simulink model "SPGF_FSK_0000_R2019b"  (R2019b)
settings: Solver=ode3  SolverName=ode4  StartTime=0.0  StopTime=1.4  FixedStep=50e-6/50  RelTol=1e-3  EnableMultiTasking=on
undefined symbols (not defined in the file): D11, Delta
libraries: powerlib x2544, powerlib_meascontrol x204, simulink x24
(part 7 of 33)

== system SPGF_FSK_0000_R2019b/W60 ==
  DPL : Subsystem  Commented=on  mask{N=6, Frequency=[50], R_matrix=[0.347601410823579 0.0494303286168989 0.0494305228057156 0.0494305228057156 0.0494305228057156 0.0494305228057156;0.0494303286168989 0.63357380919679 0.0494305228057156 0.0494305228057156 0.0494305228057156 0.0494305228057156;0.0494305228057156 0.0494305228057156 0.347602052073771 0.0494309698670905 0.0494311641268522 0.0494311641268522;0.0494305228057156 0.0494305228057156 0.0494309698670905 0.633574450446981 0.0494311641268522 0.0494311641268522;0.0494305228057156 0.0494305228057156 0.0494311641268522 0.0494311641268522 0.347602052073771 0.0494309698670905;0.0494305228057156 0.0494305228057156 0.0494311641268522 0.0494311641268522 0.0494309698670905 0.633574450446981], L_matrix=[0.00260859879857304 0.00242332383525137 0.00221745883616686 0.00221745883616686 0.00221745883616686 0.00221745883616686;0.00242332383525137 0.00242198857850016 0.00221745883616686 0.00221745883616686 0.00221745883616686 0.00221745883616686;0.00221745883616686 0.00221745883616686 0.00253519514382882 0.00234992018050715 0.00223977112704788 0.00223977112704788;0.00221745883616686 0.00221745883616686 0.00234992018050715 0.00234858492375594 0.00223977112704788 0.00223977112704788;0.00221745883616686 0.00221745883616686 0.00223977112704788 0.00223977112704788 0.00253519514382882 0.00234992018050715;0.00221745883616686 0.00221745883616686 0.00223977112704788 0.00223977112704788 0.00234992018050715 0.00234858492375594], C_matrix=[1.90757475136094e-07 -1.90757475136094e-07 0 0 0 0;-1.90757475136094e-07 3.66052807704686e-07 0 0 0 0;0 0 1.90757475136094e-07 -1.90757475136094e-07 0 0;0 0 -1.90757475136094e-07 3.66052807704686e-07 0 0;0 0 0 0 1.90757475136094e-07 -1.90757475136094e-07;0 0 0 0 -1.90757475136094e-07 3.66052807704686e-07], Rg_matrix=[834331.357019417 -834331.357019417 Inf Inf Inf -Inf;-834331.357019417 434786.838789375 Inf Inf Inf -Inf;Inf Inf 834331.357019417 -834331.357019417 Inf -Inf;Inf Inf -834331.357019417 434786.838789375 Inf -Inf;Inf Inf Inf Inf 834331.357019417 -834331.357019417;Inf Inf Inf Inf -834331.357019417 434786.838789375], LineLength=[0.8]}
      mask prompts: N "Number of phases [N]"; Frequency "Frequency used for rlc specification [Hz]:"; R_matrix "Resistance per unit length [Ohms/km] NxN matrix"; L_matrix "Inductance per unit length [H/km] NxN matrix"; C_matrix "Capacitance per unit length [F/km] NxN matrix"; Rg_matrix "Resistance shunt matrix 6*6 [Ohm*km]"; LineLength "Line Length(km)"
      mask init:
      | % Rloss=1/(2*pi*Frequency*C_matrix(1,1)*TangLoss);
      | Rg_matrix=Rg_matrix./LineLength;
      mask Display:
      | port_label('lconn',1,'A');
      | port_label('lconn',2,'B');
      | port_label('lconn',3,'C');
      | 
      | port_label('rconn',1,'a');
      | port_label('rconn',2,'b');
      | port_label('rconn',3,'c');
      | 
      | disp('1x95');
  Pi : Subsystem  mask{R0=0.31, X0=0.083, Cp0=0.35, tg=2, Frequency=[50], LineLength=[0.8]}
      mask prompts: R0 "Удельное активное сопротивление, Ом/км"; X0 "Удельное индуктивное сопротивление, Ом/км"; Cp0 "Удельная рабочая емкость, мкФ/км"; tg "Тангенс диэлектрических потерь, %"; Frequency "Частота сети, Гц"; LineLength "Длина линии, км"
      mask init:
      | R=R0*LineLength;
      | L=X0*LineLength/(2*pi*Frequency);
      | Cp=Cp0*LineLength*1e-6;
      | Cmf=0.1525*Cp;
      | Cfg=0.56*Cp;
      | tg_pu=tg/100;
      | 
      | Rmf=1/(Cmf*2*pi*Frequency*tg_pu);
      | Rfg=1/(Cfg*2*pi*Frequency*tg_pu);
      mask Display:
      | port_label('lconn',1,'A');
      | port_label('lconn',2,'B');
      | port_label('lconn',3,'C');
      | 
      | port_label('rconn',1,'a');
      | port_label('rconn',2,'b');
      | port_label('rconn',3,'c');
      | 
      | disp('1x95');
  Q : Subsystem
  concentrated : Subsystem  Commented=on  mask{N=6, Frequency=[50], R_matrix=[0.347601410823579 0.0494303286168989 0.0494305228057156 0.0494305228057156 0.0494305228057156 0.0494305228057156;0.0494303286168989 0.63357380919679 0.0494305228057156 0.0494305228057156 0.0494305228057156 0.0494305228057156;0.0494305228057156 0.0494305228057156 0.347602052073771 0.0494309698670905 0.0494311641268522 0.0494311641268522;0.0494305228057156 0.0494305228057156 0.0494309698670905 0.633574450446981 0.0494311641268522 0.0494311641268522;0.0494305228057156 0.0494305228057156 0.0494311641268522 0.0494311641268522 0.347602052073771 0.0494309698670905;0.0494305228057156 0.0494305228057156 0.0494311641268522 0.0494311641268522 0.0494309698670905 0.633574450446981], L_matrix=[0.00260859879857304 0.00242332383525137 0.00221745883616686 0.00221745883616686 0.00221745883616686 0.00221745883616686;0.00242332383525137 0.00242198857850016 0.00221745883616686 0.00221745883616686 0.00221745883616686 0.00221745883616686;0.00221745883616686 0.00221745883616686 0.00253519514382882 0.00234992018050715 0.00223977112704788 0.00223977112704788;0.00221745883616686 0.00221745883616686 0.00234992018050715 0.00234858492375594 0.00223977112704788 0.00223977112704788;0.00221745883616686 0.00221745883616686 0.00223977112704788 0.00223977112704788 0.00253519514382882 0.00234992018050715;0.00221745883616686 0.00221745883616686 0.00223977112704788 0.00223977112704788 0.00234992018050715 0.00234858492375594], C_matrix=[1.90757475136094e-07 -1.90757475136094e-07 0 0 0 0;-1.90757475136094e-07 3.66052807704686e-07 0 0 0 0;0 0 1.90757475136094e-07 -1.90757475136094e-07 0 0;0 0 -1.90757475136094e-07 3.66052807704686e-07 0 0;0 0 0 0 1.90757475136094e-07 -1.90757475136094e-07;0 0 0 0 -1.90757475136094e-07 3.66052807704686e-07], Rg_matrix=[834331.357019417 -834331.357019417 Inf Inf Inf -Inf;-834331.357019417 434786.838789375 Inf Inf Inf -Inf;Inf Inf 834331.357019417 -834331.357019417 Inf -Inf;Inf Inf -834331.357019417 434786.838789375 Inf -Inf;Inf Inf Inf Inf 834331.357019417 -834331.357019417;Inf Inf Inf Inf -834331.357019417 434786.838789375], LineLength=[0.8]}
      mask prompts: N "Number of phases [N]"; Frequency "Frequency [Hz]:"; R_matrix "Resistance matrix 6*6 [Ohm/km]"; L_matrix "Inductance matrix 6*6 [H/km]"; C_matrix "Capacitance matrix 6*6 [F/km]"; Rg_matrix "Resistance shunt matrix 6*6 [Ohm*km]"; LineLength "Line Length(km)"
      mask init: same as SPGF_FSK_0000_R2019b/W11/concentrated
      mask Display:
      | port_label('lconn',1,'A');
      | port_label('lconn',2,'B');
      | port_label('lconn',3,'C');
      | 
      | port_label('rconn',1,'a');
      | port_label('rconn',2,'b');
      | port_label('rconn',3,'c');
      | 
      | disp('1x95');
  a : PMIOPort  Side=Right
  b : PMIOPort  Port=2  Side=Right
  c : PMIOPort  Port=3  Side=Right
  A : PMIOPort  Port=4  Side=Left
  B : PMIOPort  Port=5  Side=Left
  C : PMIOPort  Port=6  Side=Left
  connections:
  Pi/RConn2 -- Q/LConn2 -- concentrated/RConn2 -- DPL/RConn2
  Pi/RConn1 -- Q/LConn1 -- concentrated/RConn1 -- DPL/RConn1
  Pi/RConn3 -- Q/LConn3 -- concentrated/RConn3 -- DPL/RConn3
  Q/RConn2 -- b/RConn1
  Q/RConn1 -- a/RConn1
  Q/RConn3 -- c/RConn1
  DPL/LConn3 -- C/RConn1 -- Pi/LConn3 -- concentrated/LConn3
  concentrated/LConn2 -- B/RConn1 -- Pi/LConn2 -- DPL/LConn2
  concentrated/LConn1 -- A/RConn1 -- Pi/LConn1 -- DPL/LConn1

== system SPGF_FSK_0000_R2019b/W61 ==
  Q : Subsystem
  a : PMIOPort  Side=Right
  b : PMIOPort  Port=2  Side=Right
  c : PMIOPort  Port=3  Side=Right
  A : PMIOPort  Port=4  Side=Left
  B : PMIOPort  Port=5  Side=Left
  C : PMIOPort  Port=6  Side=Left
  connections:
  Q/RConn3 -- c/RConn1
  Q/RConn1 -- a/RConn1
  Q/RConn2 -- b/RConn1
  Q/LConn3 -- C/RConn1
  Q/LConn1 -- A/RConn1
  Q/LConn2 -- B/RConn1

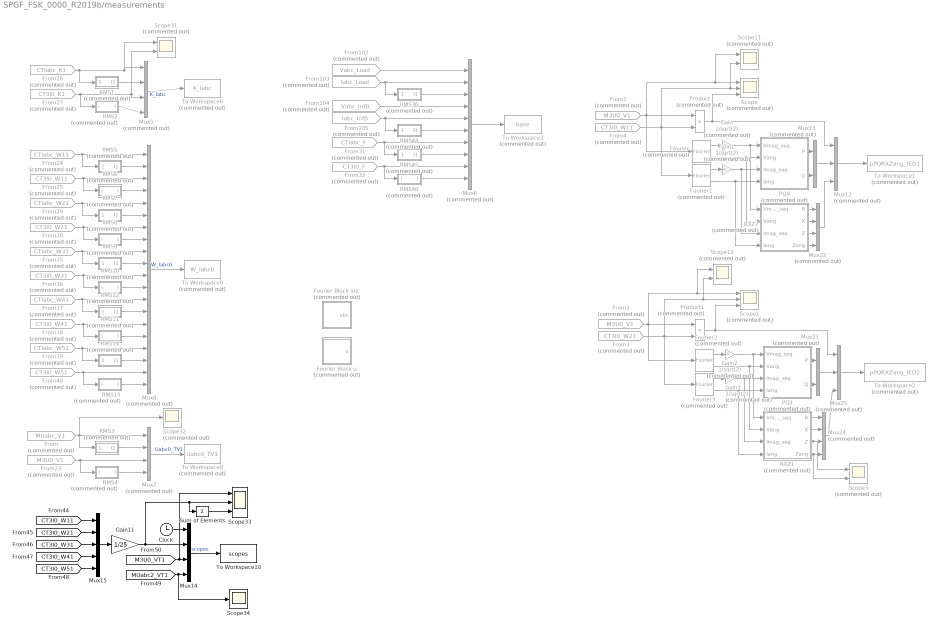
== system SPGF_FSK_0000_R2019b/measurements ==
  Clock : Clock
  Fourier{,1..3} (4 alike) : powerlib_meascontrol/Measurements/Fourier  Commented=on  Freq=50  n=1  InInit=[0, 0]  Ts=FTime
  Fourier Block abc : Subsystem  Commented=on
  Fourier Block u : Subsystem  Commented=on
  From : From  Commented=on  GotoTag=MUabc_V1  TagVisibility=global
  From1 : From  Commented=on  GotoTag=M3U0_V1  TagVisibility=global
  From102 : From  Commented=on  GotoTag=Vabc_Load  TagVisibility=global
  From103 : From  Commented=on  GotoTag=Iabc_Load  TagVisibility=global
  From104 : From  Commented=on  GotoTag=Vabc_InfB  TagVisibility=global
  From105 : From  Commented=on  GotoTag=Iabc_InfB  TagVisibility=global
  From2 : From  Commented=on  GotoTag=M3U0_V1  TagVisibility=global
  From23 : From  Commented=on  GotoTag=M3U0_V1  TagVisibility=global
  From24 : From  Commented=on  GotoTag=CTIabc_W11  TagVisibility=global
  From25 : From  Commented=on  GotoTag=CT3I0_W11  TagVisibility=global
  From26 : From  Commented=on  GotoTag=CTIabc_K1  TagVisibility=global
  From27 : From  Commented=on  GotoTag=CT3I0_K1  TagVisibility=global
  From29 : From  Commented=on  GotoTag=CTIabc_W21  TagVisibility=global
  From3 : From  Commented=on  GotoTag=CT3I0_W21  TagVisibility=global
  From30 : From  Commented=on  GotoTag=CT3I0_W21  TagVisibility=global
  From31 : From  Commented=on  GotoTag=CTIabc_F  TagVisibility=global
  From32 : From  Commented=on  GotoTag=CT3I0_F  TagVisibility=global
  From35 : From  Commented=on  GotoTag=CTIabc_W31  TagVisibility=global
  From36 : From  Commented=on  GotoTag=CT3I0_W31  TagVisibility=global
  From37 : From  Commented=on  GotoTag=CTIabc_W41  TagVisibility=global
  From38 : From  Commented=on  GotoTag=CT3I0_W41  TagVisibility=global
  From39 : From  Commented=on  GotoTag=CTIabc_W51  TagVisibility=global
  From4 : From  Commented=on  GotoTag=CT3I0_W11  TagVisibility=global
  From40 : From  Commented=on  GotoTag=CT3I0_W51  TagVisibility=global
  Gain{,1..3} (4 alike) : Gain  Commented=on  Gain=1/sqrt(2)
  Gain11 : Gain  Gain=1/25
  Mux12 : Mux  Commented=on  Inputs=3
  Mux13 : Mux  Commented=on  Inputs=2
  Mux14 : Mux
  Mux15 : Mux  Inputs=5
  Mux{5,7,22,24} (4 alike) : Mux  Commented=on
  Mux23 : Mux  Commented=on  Inputs=2
  Mux25 : Mux  Commented=on  Inputs=3
  Mux6 : Mux  Commented=on  Inputs=10
  Mux8 : Mux  Commented=on  Inputs=20
  PQ1 : Subsystem  Commented=on
  PQ8 : Subsystem  Commented=on
  Product : Product  Commented=on
  Product1 : Product  Commented=on
  RMS1 : Subsystem  Commented=on
  RMS10 : Subsystem  Commented=on
  RMS11 : Subsystem  Commented=on
  RMS12 : Subsystem  Commented=on
  RMS13 : Subsystem  Commented=on
  RMS14 : Subsystem  Commented=on
  RMS2 : Subsystem  Commented=on
  RMS3 : Subsystem  Commented=on
  RMS36 : Subsystem  Commented=on
  RMS4 : Subsystem  Commented=on
  RMS44 : Subsystem  Commented=on
  RMS45 : Subsystem  Commented=on
  RMS46 : Subsystem  Commented=on
  RMS5 : Subsystem  Commented=on
  RMS6 : Subsystem  Commented=on
  RMS7 : Subsystem  Commented=on
  RMS8 : Subsystem  Commented=on
  RMS9 : Subsystem  Commented=on
  RXZ1 : Subsystem  Commented=on
  RXZ7 : Subsystem  Commented=on
  Scope : Scope  Commented=on  NumInputPorts=3
  Scope1 : Scope  Commented=on  NumInputPorts=3
  Scope{3,11..12,31} (4 alike) : Scope  Commented=on  NumInputPorts=2
  Scope32 : Scope  Commented=on
  Scope33 : Scope  NumInputPorts=3
  Scope34 : Scope
  Sum of Elements : Sum  Inputs=+
  To Workspace1 : ToWorkspace  Commented=on  VariableName=pPQRXZang_IED1  SampleTime=-1
      settings: Save2DSignal=2-D array (concatenate along first dimension)
  To Workspace10 : ToWorkspace  VariableName=scopes  SampleTime=-1
      settings: Save2DSignal=2-D array (concatenate along first dimension)
  To Workspace2 : ToWorkspace  Commented=on  VariableName=pPQRXZang_IED2  SampleTime=-1
      settings: Save2DSignal=2-D array (concatenate along first dimension)
  To Workspace3 : ToWorkspace  Commented=on  VariableName=base  SaveFormat=Structure With Time  SampleTime=-1
      settings: Save2DSignal=2-D array (concatenate along first dimension)
  To Workspace6 : ToWorkspace  Commented=on  VariableName=K_Iabc  SampleTime=-1
      settings: Save2DSignal=2-D array (concatenate along first dimension)
  To Workspace8 : ToWorkspace  Commented=on  VariableName=Uabc0_TV1  SampleTime=-1
      settings: Save2DSignal=2-D array (concatenate along first dimension)
  To Workspace9 : ToWorkspace  Commented=on  VariableName=W_Iabc0  SampleTime=-1
      settings: Save2DSignal=2-D array (concatenate along first dimension)
  wires:
  From103/1 -> Mux6/2, RMS36/1(abc)
  From102/1 -> Mux6/1
  From104/1 -> Mux6/4
  From105/1 -> Mux6/5, RMS44/1(abc)
  From31/1 -> Mux6/7, RMS45/1(abc)
  From32/1 -> Mux6/9, RMS46/1(i)
  RMS36/1(I1) -> Mux6/3
  Mux6/1 -> To Workspace3/1
  RMS44/1(I1) -> Mux6/6
  RMS45/1(I1) -> Mux6/8
  RMS46/1(I) -> Mux6/10
  From4/1 -> Scope11/2, Scope/2, Fourier1/1, Product/2
  Product/1 -> Scope/3, Mux12/1
  Product1/1 -> Scope1/3, Mux25/1
  RXZ7/1(R) -> Mux22/1
  PQ8/2(Q) -> Mux13/2
  PQ8/1(P) -> Mux13/1
  RXZ7/2(X) -> Mux22/2
  RXZ7/4(Zang) -> Mux22/4
  Fourier/1 -> Gain/1
  Fourier1/2 -> RXZ7/4(Iang), PQ8/4(Iang)
  RXZ7/3(Z) -> Mux22/3
  Fourier1/1 -> Gain1/1
  Fourier/2 -> PQ8/2(Vang), RXZ7/2(Vang)
  Mux12/1 -> To Workspace1/1
  Gain/1 -> PQ8/1(Vmag_seq), RXZ7/1(Vmag_seq)
  Gain1/1 -> RXZ7/3(Imag_seq), PQ8/3(Imag_seq)
  Mux13/1 -> Mux12/2
  Mux22/1 -> Mux12/3
  From3/1 -> Scope1/2, Scope12/2, Fourier3/1, Product1/2
  From2/1 -> Scope12/1, Scope1/1, Fourier2/1, Product1/1
  RXZ1/1(R) -> Mux24/1
  PQ1/2(Q) -> Mux23/2
  PQ1/1(P) -> Mux23/1
  RXZ1/2(X) -> Mux24/2
  RXZ1/4(Zang) -> Scope3/2, Mux24/4
  Fourier2/1 -> Gain2/1
  Fourier3/2 -> PQ1/4(Iang), RXZ1/4(Iang)
  RXZ1/3(Z) -> Scope3/1, Mux24/3
  Fourier3/1 -> Gain3/1
  Fourier2/2 -> RXZ1/2(Vang), PQ1/2(Vang)
  Gain2/1 -> RXZ1/1(Vmag_seq), PQ1/1(Vmag_seq)
  Gain3/1 -> PQ1/3(Imag_seq), RXZ1/3(Imag_seq)
  Mux23/1 -> Mux25/2
  Mux24/1 -> Mux25/3
  Mux25/1 -> To Workspace2/1
  From1/1 -> Scope11/1, Scope/1, Fourier/1, Product/1
  From27/1 -> Scope31/2, Mux5/3, RMS2/1(i)
  From26/1 -> Scope31/1, Mux5/1, RMS1/1(abc)
  RMS1/1(I1) -> Mux5/2
  RMS2/1(I) -> Mux5/4
  Mux5/1 -> To Workspace6/1  "K_Iabc"
  Mux7/1 -> To Workspace8/1  "Uabc0_TV1"
  RMS4/1(I) -> Mux7/4
  RMS3/1(I1) -> Mux7/2
  From/1 -> Mux7/1, Scope32/1, RMS3/1(abc)
  From23/1 -> Mux7/3, RMS4/1(i)
  Mux8/1 -> To Workspace9/1  "W_Iabc0"
  RMS6/1(I) -> Mux8/4
  RMS5/1(I1) -> Mux8/2
  From24/1 -> RMS5/1(abc), Mux8/1
  From25/1 -> RMS6/1(i), Mux8/3
  From30/1 -> Mux8/7, RMS8/1(i)
  From29/1 -> Mux8/5, RMS7/1(abc)
  RMS7/1(I1) -> Mux8/6
  RMS8/1(I) -> Mux8/8
  RMS10/1(I) -> Mux8/12
  RMS9/1(I1) -> Mux8/10
  From35/1 -> Mux8/9, RMS9/1(abc)
  From36/1 -> Mux8/11, RMS10/1(i)
  From38/1 -> Mux8/15, RMS11/1(i)
  From37/1 -> Mux8/13, RMS12/1(abc)
  RMS12/1(I1) -> Mux8/14
  RMS11/1(I) -> Mux8/16
  RMS13/1(I) -> Mux8/20
  RMS14/1(I1) -> Mux8/18
  From39/1 -> Mux8/17, RMS14/1(abc)
  From40/1 -> Mux8/19, RMS13/1(i)
  Mux14/1 -> To Workspace10/1  "scopes"
  [CT3I0_W11] -> Mux15/1
  [CT3I0_W21] -> Mux15/2
  [CT3I0_W31] -> Mux15/3
  [CT3I0_W41] -> Mux15/4
  [CT3I0_W51] -> Mux15/5
  Mux15/1 -> Gain11/1
  Gain11/1 -> Mux14/2, Sum of Elements/1, Scope33/2
  [M3U0_VT1] -> Mux14/3, Scope33/1
  [MUabc2_VT1] -> Scope34/1, Mux14/4
  Clock/1 -> Mux14/1
  Sum of Elements/1 -> Scope33/3

== system SPGF_FSK_0000_R2019b/Feed/Q ==
  breaker : Subsystem  Commented=on  mask{SwitchA=off, SwitchB=off, SwitchC=off, InitialStatus=[1 1 1], BreakerResistance=0.0001, SnubberResistance=1e6, SnubberCapacitance=inf, TransitionTimes=[0.5 0.7], ShiftTimes=[0 0 0]}
      mask prompts: SwitchA "Switching of phase A"; SwitchB "Switching of phase B"; SwitchC "Switching of phase C"; InitialStatus "Initial status of phase breaker [A, B, C]"; BreakerResistance "Breaker resistance Ron (ohms) :"; SnubberResistance "Snubbers resistance Rp (ohms) :"; SnubberCapacitance "Snubbers capacitance Cp (F) :"; TransitionTimes "Transition times (s) :"; ShiftTimes "Time differences for switch [tA, tB, tC] (s) :"
      mask init:
      | SwitchA = double(SwitchA);
      | SwitchB = double(SwitchB);
      | SwitchC = double(SwitchC);
      | SwitchStatusA(1) = double((logical(InitialStatus(1))));
      | SwitchStatusB(1) = double((logical(InitialStatus(2))));
      | SwitchStatusC(1) = double((logical(InitialStatus(3))));
      | for i=1:length(TransitionTimes)
      |     SwitchStatusA(i+1) = double(~(logical(SwitchStatusA(i))));
      |     SwitchStatusB(i+1) = double(~(logical(SwitchStatusB(i))));
      |     SwitchStatusC(i+1) = double(~(logical(SwitchStatusC(i))));
      | end
      | SwitchTimesA = [0,TransitionTimes+ShiftTimes(1)];
      | SwitchTimesB = [0,TransitionTimes+ShiftTimes(2)];
      | SwitchTimesC = [0,TransitionTimes+ShiftTimes(3)];
      mask Display:
      | % port_label('input',1,'Iabc');
      | 
      | port_label('lconn',1,'A');
      | port_label('lconn',2,'B');
      | port_label('lconn',3,'C');
      | 
      | port_label('rconn',1,'a');
      | port_label('rconn',2,'b');
      | port_label('rconn',3,'c');
      | 
      | disp('   Q    ');
  meas : Subsystem
  shunt : Subsystem
  A : PMIOPort  Side=Right
  B : PMIOPort  Port=2  Side=Right
  C : PMIOPort  Port=3  Side=Right
  a : PMIOPort  Port=4  Side=Left
  b : PMIOPort  Port=5  Side=Left
  c : PMIOPort  Port=6  Side=Left
  connections:
  breaker/RConn1 -- meas/LConn1 -- shunt/RConn1
  breaker/RConn2 -- meas/LConn2 -- shunt/RConn2
  shunt/RConn3 -- breaker/RConn3 -- meas/LConn3
  shunt/LConn3 -- C/RConn1 -- breaker/LConn3
  shunt/LConn1 -- A/RConn1 -- breaker/LConn1
  shunt/LConn2 -- B/RConn1 -- breaker/LConn2
  meas/RConn1 -- a/RConn1
  meas/RConn2 -- b/RConn1
  meas/RConn3 -- c/RConn1

== system SPGF_FSK_0000_R2019b/Harmonic/Fourier Block1 ==
  in : Inport
  Display : Display
  Fourier : powerlib_meascontrol/Measurements/Fourier  Freq=50  n=1  InInit=[0, 0]  Ts=0
  Fourier1 : powerlib_meascontrol/Measurements/Fourier  Freq=50  n=2  InInit=[0, 0]  Ts=0
  Fourier2 : powerlib_meascontrol/Measurements/Fourier  Freq=50  n=3  InInit=[0, 0]  Ts=0
  Fourier3 : powerlib_meascontrol/Measurements/Fourier  Freq=50  n=5  InInit=[0, 0]  Ts=0
  Fourier4 : powerlib_meascontrol/Measurements/Fourier  Freq=50  n=7  InInit=[0, 0]  Ts=0
  Fourier5 : powerlib_meascontrol/Measurements/Fourier  Freq=50  n=9  InInit=[0, 0]  Ts=0
  Fourier6 : powerlib_meascontrol/Measurements/Fourier  Freq=50  n=11  InInit=[0, 0]  Ts=0
  Fourier7 : powerlib_meascontrol/Measurements/Fourier  Freq=50  n=13  InInit=[0, 0]  Ts=0
  Fourier8 : powerlib_meascontrol/Measurements/Fourier  Freq=50  n=15  InInit=[0, 0]  Ts=0
  Fourier9 : powerlib_meascontrol/Measurements/Fourier  Freq=50  n=17  InInit=[0, 0]  Ts=0
  Mux : Mux  Inputs=10
  Scope{2..11} (10 alike) : Scope
  Terminator{,1..9} (10 alike) : Terminator
  wires:
  Mux/1 -> Display/1
  Fourier5/1 -> Scope7/1, Mux/6
  Fourier4/1 -> Scope6/1, Mux/5
  Fourier3/1 -> Scope5/1, Mux/4
  in/1 -> Fourier/1, Fourier1/1, Fourier2/1, Fourier3/1, Fourier4/1, Fourier5/1, Fourier6/1, Fourier7/1, Fourier8/1, Fourier9/1
  Fourier1/1 -> Mux/2, Scope3/1
  Fourier9/2 -> Terminator9/1
  Fourier2/1 -> Scope4/1, Mux/3
  Fourier/1 -> Mux/1, Scope2/1
  Fourier3/2 -> Terminator5/1
  Fourier4/2 -> Terminator4/1
  Fourier5/2 -> Terminator3/1
  Fourier1/2 -> Terminator1/1
  Fourier/2 -> Terminator2/1
  Fourier8/2 -> Terminator6/1
  Fourier6/2 -> Terminator8/1
  Fourier7/2 -> Terminator7/1
  Fourier2/2 -> Terminator/1
  Fourier9/1 -> Scope11/1, Mux/10
  Fourier6/1 -> Scope8/1, Mux/7
  Fourier8/1 -> Scope10/1, Mux/9
  Fourier7/1 -> Scope9/1, Mux/8

== system SPGF_FSK_0000_R2019b/Harmonic/Fourier Block2 ==
  in : Inport
  Display : Display
  Fourier : powerlib_meascontrol/Measurements/Fourier  Freq=50  n=1  InInit=[0, 0]  Ts=0
  Fourier1 : powerlib_meascontrol/Measurements/Fourier  Freq=50  n=2  InInit=[0, 0]  Ts=0
  Fourier2 : powerlib_meascontrol/Measurements/Fourier  Freq=50  n=3  InInit=[0, 0]  Ts=0
  Fourier3 : powerlib_meascontrol/Measurements/Fourier  Freq=50  n=5  InInit=[0, 0]  Ts=0
  Fourier4 : powerlib_meascontrol/Measurements/Fourier  Freq=50  n=7  InInit=[0, 0]  Ts=0
  Fourier5 : powerlib_meascontrol/Measurements/Fourier  Freq=50  n=9  InInit=[0, 0]  Ts=0
  Fourier6 : powerlib_meascontrol/Measurements/Fourier  Freq=50  n=11  InInit=[0, 0]  Ts=0
  Fourier7 : powerlib_meascontrol/Measurements/Fourier  Freq=50  n=13  InInit=[0, 0]  Ts=0
  Fourier8 : powerlib_meascontrol/Measurements/Fourier  Freq=50  n=15  InInit=[0, 0]  Ts=0
  Fourier9 : powerlib_meascontrol/Measurements/Fourier  Freq=50  n=17  InInit=[0, 0]  Ts=0
  Mux : Mux  Inputs=10
  Scope{2..11} (10 alike) : Scope
  Terminator{,1..9} (10 alike) : Terminator
  wires:
  Fourier7/1 -> Mux/8, Scope9/1
  Fourier8/1 -> Mux/9, Scope10/1
  Fourier6/1 -> Mux/7, Scope8/1
  Fourier9/1 -> Mux/10, Scope11/1
  Fourier2/2 -> Terminator/1
  Fourier7/2 -> Terminator7/1
  Fourier6/2 -> Terminator8/1
  Fourier8/2 -> Terminator6/1
  Fourier/2 -> Terminator2/1
  Fourier1/2 -> Terminator1/1
  Fourier5/2 -> Terminator3/1
  Fourier4/2 -> Terminator4/1
  Fourier3/2 -> Terminator5/1
  Fourier/1 -> Scope2/1, Mux/1
  Fourier2/1 -> Mux/3, Scope4/1
  Fourier9/2 -> Terminator9/1
  Fourier1/1 -> Scope3/1, Mux/2
  in/1 -> Fourier9/1, Fourier8/1, Fourier7/1, Fourier6/1, Fourier5/1, Fourier4/1, Fourier3/1, Fourier2/1, Fourier1/1, Fourier/1
  Fourier3/1 -> Mux/4, Scope5/1
  Fourier4/1 -> Mux/5, Scope6/1
  Fourier5/1 -> Mux/6, Scope7/1
  Mux/1 -> Display/1

== system SPGF_FSK_0000_R2019b/Harmonic/Subsystem1 ==
  clock : Inport
  phase : Inport  Port=2
  Add : Sum
  Add1 : Sum
  Constant1 : Constant  Value=HN
  Constant2 : Constant  Value=Percent./100
  Constant3 : Constant  Value=PhaseH
  Dot Product : DotProduct  OutDataTypeStr=double  RndMeth=Nearest  InputSameDT=on
  Product15 : Product
  Trigonometric Function : Trigonometry  Operator=cos
  amp : Gain  Gain=Current*sqrt(2)
  deg2rad : Gain  Gain=pi/180
  omega1 : Gain  Gain=2*pi*Frequency
  o : Outport
  wires:
  Constant3/1 -> Add1/1
  Product15/1 -> Add/1
  deg2rad/1 -> Add/2
  phase/1 -> Add1/2
  Dot Product/1 -> o/1
  Add/1 -> Trigonometric Function/1
  Trigonometric Function/1 -> Dot Product/2
  clock/1 -> Product15/2
  Constant1/1 -> omega1/1
  Add1/1 -> deg2rad/1
  Constant2/1 -> amp/1
  amp/1 -> Dot Product/1
  omega1/1 -> Product15/1

== system SPGF_FSK_0000_R2019b/Harmonic/Subsystem2 ==
  clock : Inport
  phase : Inport  Port=2
  Add : Sum
  Add1 : Sum
  Constant1 : Constant  Value=HN
  Constant2 : Constant  Value=Percent./100
  Constant3 : Constant  Value=PhaseH
  Dot Product : DotProduct  OutDataTypeStr=double  RndMeth=Nearest  InputSameDT=on
  Product15 : Product
  Trigonometric Function : Trigonometry  Operator=cos
  amp : Gain  Gain=Current*sqrt(2)
  deg2rad : Gain  Gain=pi/180
  omega1 : Gain  Gain=2*pi*Frequency
  o : Outport
  wires:
  omega1/1 -> Product15/1
  amp/1 -> Dot Product/1
  Constant2/1 -> amp/1
  Add1/1 -> deg2rad/1
  Constant1/1 -> omega1/1
  clock/1 -> Product15/2
  Trigonometric Function/1 -> Dot Product/2
  Add/1 -> Trigonometric Function/1
  Dot Product/1 -> o/1
  phase/1 -> Add1/2
  deg2rad/1 -> Add/2
  Product15/1 -> Add/1
  Constant3/1 -> Add1/1

== system SPGF_FSK_0000_R2019b/Harmonic/Subsystem3 ==
  clock : Inport
  phase : Inport  Port=2
  Add : Sum
  Add1 : Sum
  Constant1 : Constant  Value=HN
  Constant2 : Constant  Value=Percent./100
  Constant3 : Constant  Value=PhaseH
  Dot Product : DotProduct  OutDataTypeStr=double  RndMeth=Nearest  InputSameDT=on
  Product15 : Product
  Trigonometric Function : Trigonometry  Operator=cos
  amp : Gain  Gain=Current*sqrt(2)
  deg2rad : Gain  Gain=pi/180
  omega1 : Gain  Gain=2*pi*Frequency
  o : Outport
  wires:
  omega1/1 -> Product15/1
  amp/1 -> Dot Product/1
  Constant2/1 -> amp/1
  Add1/1 -> deg2rad/1
  Constant1/1 -> omega1/1
  clock/1 -> Product15/2
  Trigonometric Function/1 -> Dot Product/2
  Add/1 -> Trigonometric Function/1
  Dot Product/1 -> o/1
  phase/1 -> Add1/2
  deg2rad/1 -> Add/2
  Product15/1 -> Add/1
  Constant3/1 -> Add1/1

== system SPGF_FSK_0000_R2019b/K1/fault ==
  Add : Sum  Inputs=+-
  Arcing : Subsystem  TreatAsAtomicUnit=on
  Constant2 : Constant  Value=FaultPhase
  Control : Product  Inputs=***
  Count Limiter : Subsystem
  Demux : Demux  Outputs=2
  Fault Interruption : Subsystem
  Fault A : Constant  Value=FaultA
  Fault A1 : Constant  Value=0
  Fault A2 : Constant  Value=LimitArcNum
  Fault A3 : Constant  Value=AddTimeDelay
  Fault B : Constant  Value=FaultB
  Fault C : Constant  Value=FaultC
  Ground1 : powerlib/Elements/Ground  LConnTagsString=a
  Ideal Switch A : powerlib/Power Electronics/Ideal Switch  Ron=FaultResistance  Lon=0  IC=0  Rs=SnubberResistance  Cs=SnubberCapacitance  Measurements=on
  Ideal Switch B : powerlib/Power Electronics/Ideal Switch  Ron=FaultResistance  Lon=0  IC=0  Rs=SnubberResistance  Cs=SnubberCapacitance  Measurements=on
  Ideal Switch C : powerlib/Power Electronics/Ideal Switch  Ron=FaultResistance  Lon=0  IC=0  Rs=SnubberResistance  Cs=SnubberCapacitance  Measurements=on
  Mux : Mux  Inputs=2
  Product : Product
  Product1 : Product
  Product2 : Product
  Rground : powerlib/Elements/Series RLC Branch  LConnTagsString=__new0  RConnTagsString=__new0  BranchType=R  Resistance=GroundResistance  Inductance=0  SetiL0=off  InitialCurrent=0  Capacitance=inf  Setx0=off  InitialVoltage=0  Measurements=None
  SW : MultiPortSwitch  DataPortForDefault=Additional data port
  SW_Limit : Switch  Criteria=u2 > Threshold  Threshold=0.5
  SW_TD : Switch  Criteria=u2 > Threshold  Threshold=0.5
  Step : Step  Time=EndFaultTime  SampleTime=0
  Step1 : Step  Time=BeginFaultTime  SampleTime=0
  Time Delay : Subsystem
  A : PMIOPort  Side=Left
  B : PMIOPort  Port=2  Side=Left
  C : PMIOPort  Port=3  Side=Left
  wires:
  Demux/2 -> [V]
  Time Delay/1(O) -> SW_TD/1
  Count Limiter/1(Count) -> Time Delay/1(Count)
  SW_TD/1 -> Count Limiter/1(I), SW_Limit/3
  Fault A3/1 -> SW_TD/2
  SW_Limit/1 -> Product2/1, Product1/1, Product/1
  Fault Interruption/1(O) -> Control/3
  Constant2/1 -> SW/1
  SW/1 -> Demux/1
  Fault A1/1 -> SW/5
  Ideal Switch A/1 -> SW/2
  Ideal Switch B/1 -> SW/3
  Ideal Switch C/1 -> SW/4
  Fault A/1 -> Product/2
  Product/1 -> Ideal Switch A/1
  Fault B/1 -> Product1/2
  Product1/1 -> Ideal Switch B/1
  Fault C/1 -> Product2/2
  Product2/1 -> Ideal Switch C/1
  Step1/1 -> Add/1
  Step/1 -> Add/2
  Add/1 -> Arcing/Enable, Control/1
  [I] -> Mux/1
  [V] -> Mux/2
  Mux/1 -> Arcing/1(I)
  Arcing/1(O) -> Control/2
  Fault A2/1 -> SW_Limit/2
  Count Limiter/2(O) -> SW_Limit/1
  Control/1 -> SW_TD/3, Time Delay/2(Control)
  Demux/1 -> [I]
  connections:
  Ideal Switch C/LConn1 -- C/RConn1
  Ideal Switch A/LConn1 -- A/RConn1
  Ideal Switch B/LConn1 -- B/RConn1
  Ideal Switch C/RConn1 -- Rground/LConn1 -- Ideal Switch A/RConn1 -- Ideal Switch B/RConn1
  Ground1/LConn1 -- Rground/RConn1

== system SPGF_FSK_0000_R2019b/K1/meas ==
  Add : Sum  Inputs=+++
  GainI : Gain
  GainI0 : Gain
  I A: : powerlib/Measurements/Current Measurement  PhasorSimulation=off  OutputType=Complex  PSBequivalent=0
  I B: : powerlib/Measurements/Current Measurement  PhasorSimulation=off  OutputType=Complex  PSBequivalent=0
  I C: : powerlib/Measurements/Current Measurement  PhasorSimulation=off  OutputType=Complex  PSBequivalent=0
  Mux : Mux  Inputs=3
  A : PMIOPort  Side=Left
  B : PMIOPort  Port=2  Side=Left
  C : PMIOPort  Port=3  Side=Left
  a : PMIOPort  Port=4  Side=Right
  b : PMIOPort  Port=5  Side=Right
  c : PMIOPort  Port=6  Side=Right
  tag scope: CT3I0_K1=global, CTIabc_K1=global
  wires:
  GainI/1 -> [CTIabc_K1]
  Mux/1 -> GainI/1
  GainI0/1 -> [CT3I0_K1]
  Add/1 -> GainI0/1
  I C:/1 -> Add/3, Mux/3
  I B:/1 -> Add/2, Mux/2
  I A:/1 -> Add/1, Mux/1
  connections:
  I B:/LConn1 -- B/RConn1
  I C:/LConn1 -- C/RConn1
  I A:/LConn1 -- A/RConn1
  a/RConn1 -- I A:/RConn1
  I B:/RConn1 -- b/RConn1
  I C:/RConn1 -- c/RConn1

== system SPGF_FSK_0000_R2019b/K2/fault ==
  Add : Sum  Inputs=+-
  Arcing : Subsystem  TreatAsAtomicUnit=on
  Constant2 : Constant  Value=FaultPhase
  Control : Product  Inputs=***
  Count Limiter : Subsystem
  Demux : Demux  Outputs=2
  Fault Interruption : Subsystem
  Fault A : Constant  Value=FaultA
  Fault A1 : Constant  Value=0
  Fault A2 : Constant  Value=LimitArcNum
  Fault A3 : Constant  Value=AddTimeDelay
  Fault B : Constant  Value=FaultB
  Fault C : Constant  Value=FaultC
  Ground1 : powerlib/Elements/Ground  LConnTagsString=a
  Ideal Switch A : powerlib/Power Electronics/Ideal Switch  Ron=FaultResistance  Lon=0  IC=0  Rs=SnubberResistance  Cs=SnubberCapacitance  Measurements=on
  Ideal Switch B : powerlib/Power Electronics/Ideal Switch  Ron=FaultResistance  Lon=0  IC=0  Rs=SnubberResistance  Cs=SnubberCapacitance  Measurements=on
  Ideal Switch C : powerlib/Power Electronics/Ideal Switch  Ron=FaultResistance  Lon=0  IC=0  Rs=SnubberResistance  Cs=SnubberCapacitance  Measurements=on
  Mux : Mux  Inputs=2
  Product : Product
  Product1 : Product
  Product2 : Product
  Rground : powerlib/Elements/Series RLC Branch  LConnTagsString=__new0  RConnTagsString=__new0  BranchType=R  Resistance=GroundResistance  Inductance=0  SetiL0=off  InitialCurrent=0  Capacitance=inf  Setx0=off  InitialVoltage=0  Measurements=None
  SW : MultiPortSwitch  DataPortForDefault=Additional data port
  SW_Limit : Switch  Criteria=u2 > Threshold  Threshold=0.5
  SW_TD : Switch  Criteria=u2 > Threshold  Threshold=0.5
  Scope : Scope
  Step : Step  Time=EndFaultTime  SampleTime=0
  Step1 : Step  Time=BeginFaultTime  SampleTime=0
  Time Delay : Subsystem
  A : PMIOPort  Side=Left
  B : PMIOPort  Port=2  Side=Left
  C : PMIOPort  Port=3  Side=Left
  wires:
  Demux/2 -> [V]
  Time Delay/1(O) -> SW_TD/1
  Count Limiter/1(Count) -> Time Delay/1(Count)
  SW_TD/1 -> Count Limiter/1(I), SW_Limit/3
  Fault A3/1 -> SW_TD/2
  SW_Limit/1 -> Product2/1, Product1/1, Product/1
  Fault Interruption/1(O) -> Control/3
  Constant2/1 -> SW/1
  SW/1 -> Demux/1
  Fault A1/1 -> SW/5
  Ideal Switch A/1 -> SW/2
  Ideal Switch B/1 -> SW/3
  Ideal Switch C/1 -> SW/4
  Fault A/1 -> Product/2
  Product/1 -> Ideal Switch A/1
  Fault B/1 -> Product1/2
  Product1/1 -> Ideal Switch B/1
  Fault C/1 -> Product2/2
  Product2/1 -> Ideal Switch C/1
  Step1/1 -> Add/1
  Step/1 -> Add/2
  Add/1 -> Arcing/Enable, Control/1
  [I] -> Mux/1
  [V] -> Mux/2
  Mux/1 -> Arcing/1(I)
  Arcing/1(O) -> Control/2
  Fault A2/1 -> SW_Limit/2
  Count Limiter/2(O) -> SW_Limit/1
  Control/1 -> SW_TD/3, Time Delay/2(Control)
  Demux/1 -> Scope/1, [I]
  connections:
  Ideal Switch C/LConn1 -- C/RConn1
  Ideal Switch A/LConn1 -- A/RConn1
  Ideal Switch B/LConn1 -- B/RConn1
  Ideal Switch C/RConn1 -- Rground/LConn1 -- Ideal Switch A/RConn1 -- Ideal Switch B/RConn1
  Ground1/LConn1 -- Rground/RConn1

== system SPGF_FSK_0000_R2019b/K2/meas ==
  Add : Sum  Inputs=+++
  GainI : Gain
  GainI0 : Gain
  I A: : powerlib/Measurements/Current Measurement  PhasorSimulation=off  OutputType=Complex  PSBequivalent=0
  I B: : powerlib/Measurements/Current Measurement  PhasorSimulation=off  OutputType=Complex  PSBequivalent=0
  I C: : powerlib/Measurements/Current Measurement  PhasorSimulation=off  OutputType=Complex  PSBequivalent=0
  Mux : Mux  Inputs=3
  A : PMIOPort  Side=Left
  B : PMIOPort  Port=2  Side=Left
  C : PMIOPort  Port=3  Side=Left
  a : PMIOPort  Port=4  Side=Right
  b : PMIOPort  Port=5  Side=Right
  c : PMIOPort  Port=6  Side=Right
  tag scope: CT3I0_K2=global, CTIabc_K2=global
  wires:
  I A:/1 -> Mux/1, Add/1
  I B:/1 -> Mux/2, Add/2
  I C:/1 -> Mux/3, Add/3
  Add/1 -> GainI0/1
  GainI0/1 -> [CT3I0_K2]
  Mux/1 -> GainI/1
  GainI/1 -> [CTIabc_K2]
  connections:
  I C:/RConn1 -- c/RConn1
  I B:/RConn1 -- b/RConn1
  a/RConn1 -- I A:/RConn1
  I A:/LConn1 -- A/RConn1
  I C:/LConn1 -- C/RConn1
  I B:/LConn1 -- B/RConn1

== system SPGF_FSK_0000_R2019b/K3/fault ==
  Add : Sum  Inputs=+-
  Arcing : Subsystem  TreatAsAtomicUnit=on
  Constant2 : Constant  Value=FaultPhase
  Control : Product  Inputs=***
  Count Limiter : Subsystem
  Demux : Demux  Outputs=2
  Fault Interruption : Subsystem
  Fault A : Constant  Value=FaultA
  Fault A1 : Constant  Value=0
  Fault A2 : Constant  Value=LimitArcNum
  Fault A3 : Constant  Value=AddTimeDelay
  Fault B : Constant  Value=FaultB
  Fault C : Constant  Value=FaultC
  Ground1 : powerlib/Elements/Ground  LConnTagsString=a
  Ideal Switch A : powerlib/Power Electronics/Ideal Switch  Ron=FaultResistance  Lon=0  IC=0  Rs=SnubberResistance  Cs=SnubberCapacitance  Measurements=on
  Ideal Switch B : powerlib/Power Electronics/Ideal Switch  Ron=FaultResistance  Lon=0  IC=0  Rs=SnubberResistance  Cs=SnubberCapacitance  Measurements=on
  Ideal Switch C : powerlib/Power Electronics/Ideal Switch  Ron=FaultResistance  Lon=0  IC=0  Rs=SnubberResistance  Cs=SnubberCapacitance  Measurements=on
  Mux : Mux  Inputs=2
  Product : Product
  Product1 : Product
  Product2 : Product
  Rground : powerlib/Elements/Series RLC Branch  LConnTagsString=__new0  RConnTagsString=__new0  BranchType=R  Resistance=GroundResistance  Inductance=0  SetiL0=off  InitialCurrent=0  Capacitance=inf  Setx0=off  InitialVoltage=0  Measurements=None
  SW : MultiPortSwitch  DataPortForDefault=Additional data port
  SW_Limit : Switch  Criteria=u2 > Threshold  Threshold=0.5
  SW_TD : Switch  Criteria=u2 > Threshold  Threshold=0.5
  Step : Step  Time=EndFaultTime  SampleTime=0
  Step1 : Step  Time=BeginFaultTime  SampleTime=0
  Time Delay : Subsystem
  A : PMIOPort  Side=Left
  B : PMIOPort  Port=2  Side=Left
  C : PMIOPort  Port=3  Side=Left
  wires:
  Demux/2 -> [V]
  Time Delay/1(O) -> SW_TD/1
  Count Limiter/1(Count) -> Time Delay/1(Count)
  SW_TD/1 -> Count Limiter/1(I), SW_Limit/3
  Fault A3/1 -> SW_TD/2
  SW_Limit/1 -> Product2/1, Product1/1, Product/1
  Fault Interruption/1(O) -> Control/3
  Constant2/1 -> SW/1
  SW/1 -> Demux/1
  Fault A1/1 -> SW/5
  Ideal Switch A/1 -> SW/2
  Ideal Switch B/1 -> SW/3
  Ideal Switch C/1 -> SW/4
  Fault A/1 -> Product/2
  Product/1 -> Ideal Switch A/1
  Fault B/1 -> Product1/2
  Product1/1 -> Ideal Switch B/1
  Fault C/1 -> Product2/2
  Product2/1 -> Ideal Switch C/1
  Step1/1 -> Add/1
  Step/1 -> Add/2
  Add/1 -> Arcing/Enable, Control/1
  [I] -> Mux/1
  [V] -> Mux/2
  Mux/1 -> Arcing/1(I)
  Arcing/1(O) -> Control/2
  Fault A2/1 -> SW_Limit/2
  Count Limiter/2(O) -> SW_Limit/1
  Control/1 -> SW_TD/3, Time Delay/2(Control)
  Demux/1 -> [I]
  connections:
  Ideal Switch C/LConn1 -- C/RConn1
  Ideal Switch A/LConn1 -- A/RConn1
  Ideal Switch B/LConn1 -- B/RConn1
  Ideal Switch C/RConn1 -- Rground/LConn1 -- Ideal Switch A/RConn1 -- Ideal Switch B/RConn1
  Ground1/LConn1 -- Rground/RConn1

== system SPGF_FSK_0000_R2019b/K3/meas ==
  Add : Sum  Inputs=+++
  GainI : Gain
  GainI0 : Gain
  I A: : powerlib/Measurements/Current Measurement  PhasorSimulation=off  OutputType=Complex  PSBequivalent=0
  I B: : powerlib/Measurements/Current Measurement  PhasorSimulation=off  OutputType=Complex  PSBequivalent=0
  I C: : powerlib/Measurements/Current Measurement  PhasorSimulation=off  OutputType=Complex  PSBequivalent=0
  Mux : Mux  Inputs=3
  A : PMIOPort  Side=Left
  B : PMIOPort  Port=2  Side=Left
  C : PMIOPort  Port=3  Side=Left
  a : PMIOPort  Port=4  Side=Right
  b : PMIOPort  Port=5  Side=Right
  c : PMIOPort  Port=6  Side=Right
  tag scope: CT3I0_K1=global, CTIabc_K1=global
  wires:
  I A:/1 -> Mux/1, Add/1
  I B:/1 -> Mux/2, Add/2
  I C:/1 -> Mux/3, Add/3
  Add/1 -> GainI0/1
  GainI0/1 -> [CT3I0_K1]
  Mux/1 -> GainI/1
  GainI/1 -> [CTIabc_K1]
  connections:
  I C:/RConn1 -- c/RConn1
  I B:/RConn1 -- b/RConn1
  a/RConn1 -- I A:/RConn1
  I A:/LConn1 -- A/RConn1
  I C:/LConn1 -- C/RConn1
  I B:/LConn1 -- B/RConn1

== system SPGF_FSK_0000_R2019b/K4/fault ==
  Add : Sum  Inputs=+-
  Arcing : Subsystem  TreatAsAtomicUnit=on
  Constant2 : Constant  Value=FaultPhase
  Control : Product  Inputs=***
  Count Limiter : Subsystem
  Demux : Demux  Outputs=2
  Fault Interruption : Subsystem
  Fault A : Constant  Value=FaultA
  Fault A1 : Constant  Value=0
  Fault A2 : Constant  Value=LimitArcNum
  Fault A3 : Constant  Value=AddTimeDelay
  Fault B : Constant  Value=FaultB
  Fault C : Constant  Value=FaultC
  Ground1 : powerlib/Elements/Ground  LConnTagsString=a
  Ideal Switch A : powerlib/Power Electronics/Ideal Switch  Ron=FaultResistance  Lon=0  IC=0  Rs=SnubberResistance  Cs=SnubberCapacitance  Measurements=on
  Ideal Switch B : powerlib/Power Electronics/Ideal Switch  Ron=FaultResistance  Lon=0  IC=0  Rs=SnubberResistance  Cs=SnubberCapacitance  Measurements=on
  Ideal Switch C : powerlib/Power Electronics/Ideal Switch  Ron=FaultResistance  Lon=0  IC=0  Rs=SnubberResistance  Cs=SnubberCapacitance  Measurements=on
  Mux : Mux  Inputs=2
  Product : Product
  Product1 : Product
  Product2 : Product
  Rground : powerlib/Elements/Series RLC Branch  LConnTagsString=__new0  RConnTagsString=__new0  BranchType=R  Resistance=GroundResistance  Inductance=0  SetiL0=off  InitialCurrent=0  Capacitance=inf  Setx0=off  InitialVoltage=0  Measurements=None
  SW : MultiPortSwitch  DataPortForDefault=Additional data port
  SW_Limit : Switch  Criteria=u2 > Threshold  Threshold=0.5
  SW_TD : Switch  Criteria=u2 > Threshold  Threshold=0.5
  Step : Step  Time=EndFaultTime  SampleTime=0
  Step1 : Step  Time=BeginFaultTime  SampleTime=0
  Time Delay : Subsystem
  A : PMIOPort  Side=Left
  B : PMIOPort  Port=2  Side=Left
  C : PMIOPort  Port=3  Side=Left
  wires:
  Demux/2 -> [V]
  Time Delay/1(O) -> SW_TD/1
  Count Limiter/1(Count) -> Time Delay/1(Count)
  SW_TD/1 -> Count Limiter/1(I), SW_Limit/3
  Fault A3/1 -> SW_TD/2
  SW_Limit/1 -> Product2/1, Product1/1, Product/1
  Fault Interruption/1(O) -> Control/3
  Constant2/1 -> SW/1
  SW/1 -> Demux/1
  Fault A1/1 -> SW/5
  Ideal Switch A/1 -> SW/2
  Ideal Switch B/1 -> SW/3
  Ideal Switch C/1 -> SW/4
  Fault A/1 -> Product/2
  Product/1 -> Ideal Switch A/1
  Fault B/1 -> Product1/2
  Product1/1 -> Ideal Switch B/1
  Fault C/1 -> Product2/2
  Product2/1 -> Ideal Switch C/1
  Step1/1 -> Add/1
  Step/1 -> Add/2
  Add/1 -> Arcing/Enable, Control/1
  [I] -> Mux/1
  [V] -> Mux/2
  Mux/1 -> Arcing/1(I)
  Arcing/1(O) -> Control/2
  Fault A2/1 -> SW_Limit/2
  Count Limiter/2(O) -> SW_Limit/1
  Control/1 -> SW_TD/3, Time Delay/2(Control)
  Demux/1 -> [I]
  connections:
  Ideal Switch C/LConn1 -- C/RConn1
  Ideal Switch A/LConn1 -- A/RConn1
  Ideal Switch B/LConn1 -- B/RConn1
  Ideal Switch C/RConn1 -- Rground/LConn1 -- Ideal Switch A/RConn1 -- Ideal Switch B/RConn1
  Ground1/LConn1 -- Rground/RConn1

== system SPGF_FSK_0000_R2019b/K4/meas ==
  Add : Sum  Inputs=+++
  GainI : Gain
  GainI0 : Gain
  I A: : powerlib/Measurements/Current Measurement  PhasorSimulation=off  OutputType=Complex  PSBequivalent=0
  I B: : powerlib/Measurements/Current Measurement  PhasorSimulation=off  OutputType=Complex  PSBequivalent=0
  I C: : powerlib/Measurements/Current Measurement  PhasorSimulation=off  OutputType=Complex  PSBequivalent=0
  Mux : Mux  Inputs=3
  A : PMIOPort  Side=Left
  B : PMIOPort  Port=2  Side=Left
  C : PMIOPort  Port=3  Side=Left
  a : PMIOPort  Port=4  Side=Right
  b : PMIOPort  Port=5  Side=Right
  c : PMIOPort  Port=6  Side=Right
  tag scope: CT3I0_K1=global, CTIabc_K1=global
  wires:
  GainI/1 -> [CTIabc_K1]
  Mux/1 -> GainI/1
  GainI0/1 -> [CT3I0_K1]
  Add/1 -> GainI0/1
  I C:/1 -> Add/3, Mux/3
  I B:/1 -> Add/2, Mux/2
  I A:/1 -> Add/1, Mux/1
  connections:
  I B:/LConn1 -- B/RConn1
  I C:/LConn1 -- C/RConn1
  I A:/LConn1 -- A/RConn1
  a/RConn1 -- I A:/RConn1
  I B:/RConn1 -- b/RConn1
  I C:/RConn1 -- c/RConn1

== system SPGF_FSK_0000_R2019b/K5/fault ==
  Add : Sum  Inputs=+-
  Arcing : Subsystem  TreatAsAtomicUnit=on
  Constant2 : Constant  Value=FaultPhase
  Control : Product  Inputs=***
  Count Limiter : Subsystem
  Demux : Demux  Outputs=2
  Fault Interruption : Subsystem
  Fault A : Constant  Value=FaultA
  Fault A1 : Constant  Value=0
  Fault A2 : Constant  Value=LimitArcNum
  Fault A3 : Constant  Value=AddTimeDelay
  Fault B : Constant  Value=FaultB
  Fault C : Constant  Value=FaultC
  Ground1 : powerlib/Elements/Ground  LConnTagsString=a
  Ideal Switch A : powerlib/Power Electronics/Ideal Switch  Ron=FaultResistance  Lon=0  IC=0  Rs=SnubberResistance  Cs=SnubberCapacitance  Measurements=on
  Ideal Switch B : powerlib/Power Electronics/Ideal Switch  Ron=FaultResistance  Lon=0  IC=0  Rs=SnubberResistance  Cs=SnubberCapacitance  Measurements=on
  Ideal Switch C : powerlib/Power Electronics/Ideal Switch  Ron=FaultResistance  Lon=0  IC=0  Rs=SnubberResistance  Cs=SnubberCapacitance  Measurements=on
  Mux : Mux  Inputs=2
  Product : Product
  Product1 : Product
  Product2 : Product
  Rground : powerlib/Elements/Series RLC Branch  LConnTagsString=__new0  RConnTagsString=__new0  BranchType=R  Resistance=GroundResistance  Inductance=0  SetiL0=off  InitialCurrent=0  Capacitance=inf  Setx0=off  InitialVoltage=0  Measurements=None
  SW : MultiPortSwitch  DataPortForDefault=Additional data port
  SW_Limit : Switch  Criteria=u2 > Threshold  Threshold=0.5
  SW_TD : Switch  Criteria=u2 > Threshold  Threshold=0.5
  Step : Step  Time=EndFaultTime  SampleTime=0
  Step1 : Step  Time=BeginFaultTime  SampleTime=0
  Time Delay : Subsystem
  A : PMIOPort  Side=Left
  B : PMIOPort  Port=2  Side=Left
  C : PMIOPort  Port=3  Side=Left
  wires:
  Demux/2 -> [V]
  Time Delay/1(O) -> SW_TD/1
  Count Limiter/1(Count) -> Time Delay/1(Count)
  SW_TD/1 -> Count Limiter/1(I), SW_Limit/3
  Fault A3/1 -> SW_TD/2
  SW_Limit/1 -> Product2/1, Product1/1, Product/1
  Fault Interruption/1(O) -> Control/3
  Constant2/1 -> SW/1
  SW/1 -> Demux/1
  Fault A1/1 -> SW/5
  Ideal Switch A/1 -> SW/2
  Ideal Switch B/1 -> SW/3
  Ideal Switch C/1 -> SW/4
  Fault A/1 -> Product/2
  Product/1 -> Ideal Switch A/1
  Fault B/1 -> Product1/2
  Product1/1 -> Ideal Switch B/1
  Fault C/1 -> Product2/2
  Product2/1 -> Ideal Switch C/1
  Step1/1 -> Add/1
  Step/1 -> Add/2
  Add/1 -> Arcing/Enable, Control/1
  [I] -> Mux/1
  [V] -> Mux/2
  Mux/1 -> Arcing/1(I)
  Arcing/1(O) -> Control/2
  Fault A2/1 -> SW_Limit/2
  Count Limiter/2(O) -> SW_Limit/1
  Control/1 -> SW_TD/3, Time Delay/2(Control)
  Demux/1 -> [I]
  connections:
  Ideal Switch C/LConn1 -- C/RConn1
  Ideal Switch A/LConn1 -- A/RConn1
  Ideal Switch B/LConn1 -- B/RConn1
  Ideal Switch C/RConn1 -- Rground/LConn1 -- Ideal Switch A/RConn1 -- Ideal Switch B/RConn1
  Ground1/LConn1 -- Rground/RConn1

== system SPGF_FSK_0000_R2019b/K5/meas ==
  Add : Sum  Inputs=+++
  GainI : Gain
  GainI0 : Gain
  I A: : powerlib/Measurements/Current Measurement  PhasorSimulation=off  OutputType=Complex  PSBequivalent=0
  I B: : powerlib/Measurements/Current Measurement  PhasorSimulation=off  OutputType=Complex  PSBequivalent=0
  I C: : powerlib/Measurements/Current Measurement  PhasorSimulation=off  OutputType=Complex  PSBequivalent=0
  Mux : Mux  Inputs=3
  A : PMIOPort  Side=Left
  B : PMIOPort  Port=2  Side=Left
  C : PMIOPort  Port=3  Side=Left
  a : PMIOPort  Port=4  Side=Right
  b : PMIOPort  Port=5  Side=Right
  c : PMIOPort  Port=6  Side=Right
  tag scope: CT3I0_K1=global, CTIabc_K1=global
  wires:
  I A:/1 -> Mux/1, Add/1
  I B:/1 -> Mux/2, Add/2
  I C:/1 -> Mux/3, Add/3
  Add/1 -> GainI0/1
  GainI0/1 -> [CT3I0_K1]
  Mux/1 -> GainI/1
  GainI/1 -> [CTIabc_K1]
  connections:
  I C:/RConn1 -- c/RConn1
  I B:/RConn1 -- b/RConn1
  a/RConn1 -- I A:/RConn1
  I A:/LConn1 -- A/RConn1
  I C:/LConn1 -- C/RConn1
  I B:/LConn1 -- B/RConn1

== system SPGF_FSK_0000_R2019b/K6/fault ==
  Add : Sum  Inputs=+-
  Arcing : Subsystem  TreatAsAtomicUnit=on
  Constant2 : Constant  Value=FaultPhase
  Control : Product  Inputs=***
  Count Limiter : Subsystem
  Demux : Demux  Outputs=2
  Fault Interruption : Subsystem
  Fault A : Constant  Value=FaultA
  Fault A1 : Constant  Value=0
  Fault A2 : Constant  Value=LimitArcNum
  Fault A3 : Constant  Value=AddTimeDelay
  Fault B : Constant  Value=FaultB
  Fault C : Constant  Value=FaultC
  Ground1 : powerlib/Elements/Ground  LConnTagsString=a
  Ideal Switch A : powerlib/Power Electronics/Ideal Switch  Ron=FaultResistance  Lon=0  IC=0  Rs=SnubberResistance  Cs=SnubberCapacitance  Measurements=on
  Ideal Switch B : powerlib/Power Electronics/Ideal Switch  Ron=FaultResistance  Lon=0  IC=0  Rs=SnubberResistance  Cs=SnubberCapacitance  Measurements=on
  Ideal Switch C : powerlib/Power Electronics/Ideal Switch  Ron=FaultResistance  Lon=0  IC=0  Rs=SnubberResistance  Cs=SnubberCapacitance  Measurements=on
  Mux : Mux  Inputs=2
  Product : Product
  Product1 : Product
  Product2 : Product
  Rground : powerlib/Elements/Series RLC Branch  LConnTagsString=__new0  RConnTagsString=__new0  BranchType=R  Resistance=GroundResistance  Inductance=0  SetiL0=off  InitialCurrent=0  Capacitance=inf  Setx0=off  InitialVoltage=0  Measurements=None
  SW : MultiPortSwitch  DataPortForDefault=Additional data port
  SW_Limit : Switch  Criteria=u2 > Threshold  Threshold=0.5
  SW_TD : Switch  Criteria=u2 > Threshold  Threshold=0.5
  Step : Step  Time=EndFaultTime  SampleTime=0
  Step1 : Step  Time=BeginFaultTime  SampleTime=0
  Time Delay : Subsystem
  A : PMIOPort  Side=Left
  B : PMIOPort  Port=2  Side=Left
  C : PMIOPort  Port=3  Side=Left
  wires:
  Demux/2 -> [V]
  Time Delay/1(O) -> SW_TD/1
  Count Limiter/1(Count) -> Time Delay/1(Count)
  SW_TD/1 -> Count Limiter/1(I), SW_Limit/3
  Fault A3/1 -> SW_TD/2
  SW_Limit/1 -> Product2/1, Product1/1, Product/1
  Fault Interruption/1(O) -> Control/3
  Constant2/1 -> SW/1
  SW/1 -> Demux/1
  Fault A1/1 -> SW/5
  Ideal Switch A/1 -> SW/2
  Ideal Switch B/1 -> SW/3
  Ideal Switch C/1 -> SW/4
  Fault A/1 -> Product/2
  Product/1 -> Ideal Switch A/1
  Fault B/1 -> Product1/2
  Product1/1 -> Ideal Switch B/1
  Fault C/1 -> Product2/2
  Product2/1 -> Ideal Switch C/1
  Step1/1 -> Add/1
  Step/1 -> Add/2
  Add/1 -> Arcing/Enable, Control/1
  [I] -> Mux/1
  [V] -> Mux/2
  Mux/1 -> Arcing/1(I)
  Arcing/1(O) -> Control/2
  Fault A2/1 -> SW_Limit/2
  Count Limiter/2(O) -> SW_Limit/1
  Control/1 -> SW_TD/3, Time Delay/2(Control)
  Demux/1 -> [I]
  connections:
  Ideal Switch C/LConn1 -- C/RConn1
  Ideal Switch A/LConn1 -- A/RConn1
  Ideal Switch B/LConn1 -- B/RConn1
  Ideal Switch C/RConn1 -- Rground/LConn1 -- Ideal Switch A/RConn1 -- Ideal Switch B/RConn1
  Ground1/LConn1 -- Rground/RConn1

== system SPGF_FSK_0000_R2019b/K6/meas ==
  Add : Sum  Inputs=+++
  GainI : Gain
  GainI0 : Gain
  I A: : powerlib/Measurements/Current Measurement  PhasorSimulation=off  OutputType=Complex  PSBequivalent=0
  I B: : powerlib/Measurements/Current Measurement  PhasorSimulation=off  OutputType=Complex  PSBequivalent=0
  I C: : powerlib/Measurements/Current Measurement  PhasorSimulation=off  OutputType=Complex  PSBequivalent=0
  Mux : Mux  Inputs=3
  A : PMIOPort  Side=Left
  B : PMIOPort  Port=2  Side=Left
  C : PMIOPort  Port=3  Side=Left
  a : PMIOPort  Port=4  Side=Right
  b : PMIOPort  Port=5  Side=Right
  c : PMIOPort  Port=6  Side=Right
  tag scope: CT3I0_K1=global, CTIabc_K1=global
  wires:
  I A:/1 -> Mux/1, Add/1
  I B:/1 -> Mux/2, Add/2
  I C:/1 -> Mux/3, Add/3
  Add/1 -> GainI0/1
  GainI0/1 -> [CT3I0_K1]
  Mux/1 -> GainI/1
  GainI/1 -> [CTIabc_K1]
  connections:
  I C:/RConn1 -- c/RConn1
  I B:/RConn1 -- b/RConn1
  a/RConn1 -- I A:/RConn1
  I A:/LConn1 -- A/RConn1
  I C:/LConn1 -- C/RConn1
  I B:/LConn1 -- B/RConn1
